simulink model "m13solm4"  (Simulink 7.7)
settings: Solver=ode45  StartTime=1  StopTime=100  FixedStep=0.001  MaxStep=0.001  MinStep=0.0001  RelTol=1e-3
undefined symbols (not defined in the file): nmax, nmax2, nmin, nmin2, seed, seed2, tc
settings Model: Creator=Esben  LastModifiedBy=Esben

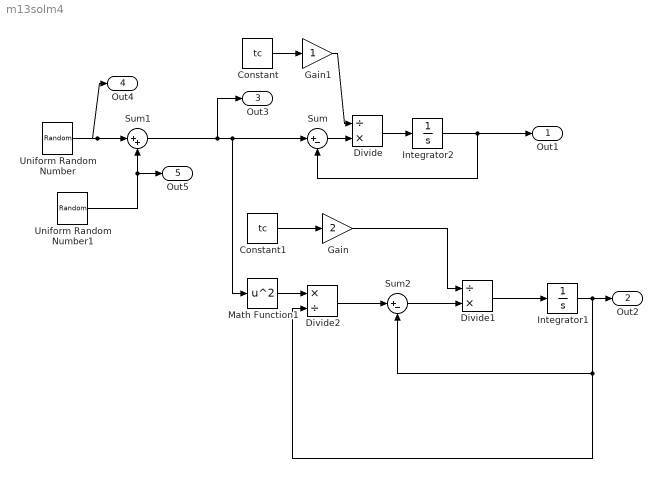
== system m13solm4 ==
  Constant : Constant  Value=tc
  Constant1 : Constant  Value=tc
  Divide : Product  Inputs=/*
  Divide1 : Product  Inputs=/*
  Divide2 : Product  Inputs=*/
  Gain : Gain  Gain=2
  Gain1 : Gain
  Integrator1 : Integrator  InitialCondition=0.0001
  Integrator2 : Integrator  InitialCondition=0.0001
  Math Function1 : Math  Operator=square  SaturateOnIntegerOverflow=on
  Sum : Sum  Inputs=|+-
  Sum1 : Sum  Inputs=|++
  Sum2 : Sum  Inputs=|+-
  Uniform Random Number : UniformRandomNumber  Minimum=nmin  Maximum=nmax  Seed=seed  SampleTime=1
  Uniform Random Number1 : UniformRandomNumber  Minimum=nmin2  Maximum=nmax2  Seed=seed2  SampleTime=1
  Out1 : Outport
  Out2 : Outport  Port=2
  Out3 : Outport  Port=3
  Out4 : Outport  Port=4
  Out5 : Outport  Port=5
  wires:
  Sum1/1 -> Sum/1, Math Function1/1, Out3/1
  Sum/1 -> Divide/2
  Constant/1 -> Gain1/1
  Divide/1 -> Integrator2/1
  Integrator2/1 -> Sum/2, Out1/1
  Constant1/1 -> Gain/1
  Divide1/1 -> Integrator1/1
  Integrator1/1 -> Sum2/2, Divide2/2, Out2/1
  Gain/1 -> Divide1/1
  Sum2/1 -> Divide1/2
  Divide2/1 -> Sum2/1
  Math Function1/1 -> Divide2/1
  Gain1/1 -> Divide/1
  Uniform Random Number1/1 -> Sum1/2, Out5/1
  Uniform Random Number/1 -> Sum1/1, Out4/1
